simulink model "w1p5_model"  (R2020a)
settings: Solver=VariableStepAuto  StartTime=0.0  StopTime=10.0  RelTol=1e-3
model workspace (MAT data in the model file):
  C = Simulink.Parameter
  C.Value = 1e-05
  C.DataType = 'auto'
  C.Dimensions = [1 1]
  R = Simulink.Parameter
  R.Value = 10
  R.DataType = 'auto'
  R.Dimensions = [1 1]
settings Model: Creator=avn19  LastModifiedBy=avn19

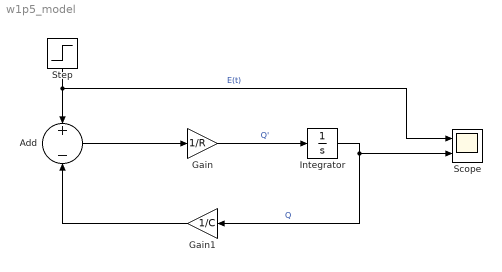
== system w1p5_model ==
  Add : Sum  Inputs=+-
  Gain : Gain  Gain=1/R
  Gain1 : Gain  Gain=1/C
  Integrator : Integrator
  Scope : Scope  NumInputPorts=2
  Step : Step  Before=2  After=9  SampleTime=0
  wires:
  Add/1 -> Gain/1
  Step/1 -> Scope/1, Add/1  "E(t)"
  Gain/1 -> Integrator/1  "Q'"
  Integrator/1 -> Gain1/1, Scope/2  "Q"
  Gain1/1 -> Add/2
